simulink model "Task35"  (R2022b)
settings: Solver=VariableStepAuto  StartTime=0.0  StopTime=10.0  RelTol=1e-3
settings Model: Creator=LOQ  LastModifiedBy=LOQ
settings OptimizationCC: ReuseModelBlockBuffer=on
settings RTWCC: GPUComputeCapability=5.0
settings ConfigComp: CovBoundaryAbsTol=1.0e-5

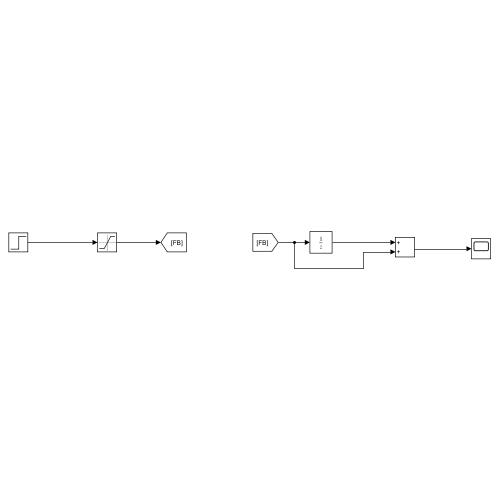
[thumbnail: Simulink's stored preview of the top-level diagram]
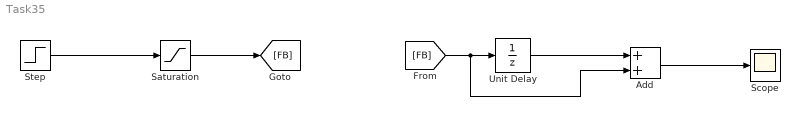
== system Task35 ==
  Add : Sum
  Saturation : Saturate  UpperLimit=10  LowerLimit=-10
  Scope : Scope
  Step : Step  After=50  SampleTime=0
  Unit Delay : UnitDelay  SampleTime=-1  HasFrameUpgradeWarning=on
  wires:
  Step/1 -> Saturation/1
  Saturation/1 -> [FB]
  [FB] -> Add/2, Unit Delay/1
  Unit Delay/1 -> Add/1
  Add/1 -> Scope/1
